simulink model "Observateur_vitesse_angulaire"  (R2022b)
settings: Solver=VariableStepAuto  StartTime=0.0  StopTime=10.0  RelTol=1e-3
undefined symbols (not defined in the file): Ld, Lp
settings Model: Creator=cheye  LastModifiedBy=cheye

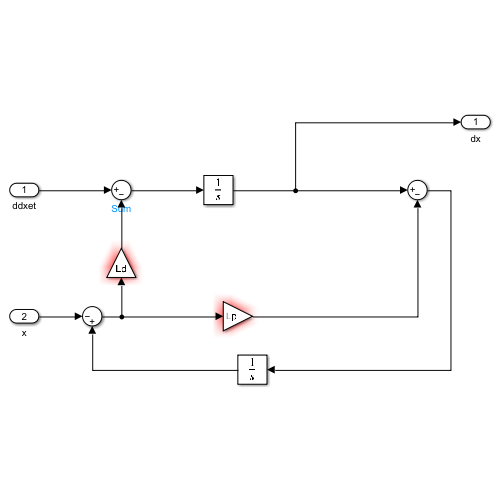
[thumbnail: Simulink's stored preview of the top-level diagram]
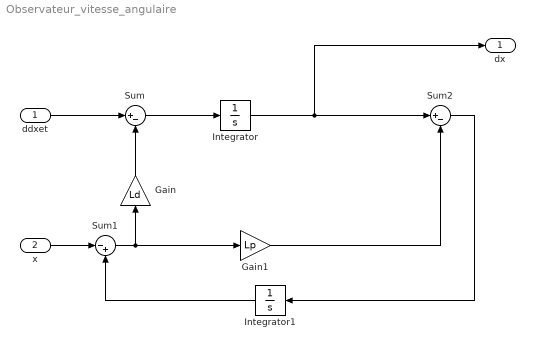
== system Observateur_vitesse_angulaire ==
  ddxet : Inport
  x : Inport  Port=2
  Gain : Gain  Gain=Ld
  Gain1 : Gain  Gain=Lp
  Integrator : Integrator
  Integrator1 : Integrator
  Sum : Sum  Inputs=|+-
  Sum1 : Sum  Inputs=|-+
  Sum2 : Sum  Inputs=|+-
  dx : Outport
  wires:
  ddxet/1 -> Sum/1
  x/1 -> Sum1/1
  Sum/1 -> Integrator/1
  Integrator1/1 -> Sum1/2
  Integrator/1 -> dx/1, Sum2/1
  Sum1/1 -> Gain/1, Gain1/1
  Gain/1 -> Sum/2
  Gain1/1 -> Sum2/2
  Sum2/1 -> Integrator1/1
